simulink model "Tavola3_SIM"  (R2018b)
settings: Solver=VariableStepAuto  StartTime=0.0  StopTime=50  RelTol=1e-3
values from neighbouring files (symbols this model uses):
  cond_iniziali = [0,0,0,10*pi/180,0,5,0]    [tavola3_LAST.m]
  cz = R    (= 0.25)    [tavola3_COORDINATEPENDOLO.m]    (also in tavola3_LAST.m; tavola3_x3x6.m; zero_dyn_x3x6.m)
  K1 = place(A_min,B_min,poles)    [tavola3_COORDINATEPENDOLO.m]    (also in tavola3_LAST.m; tavola3_x3x6.m)
  K2 = place(A_min2,B_min2,poles)    [tavola3_COORDINATEPENDOLO.m]    (also in tavola3_LAST.m; tavola3_x3x6.m)
undefined symbols (not defined in the file or in its folder): sigbuilder_block
libraries: simulink x1
settings Model: Creator=Utente  LastModifiedBy=Utente

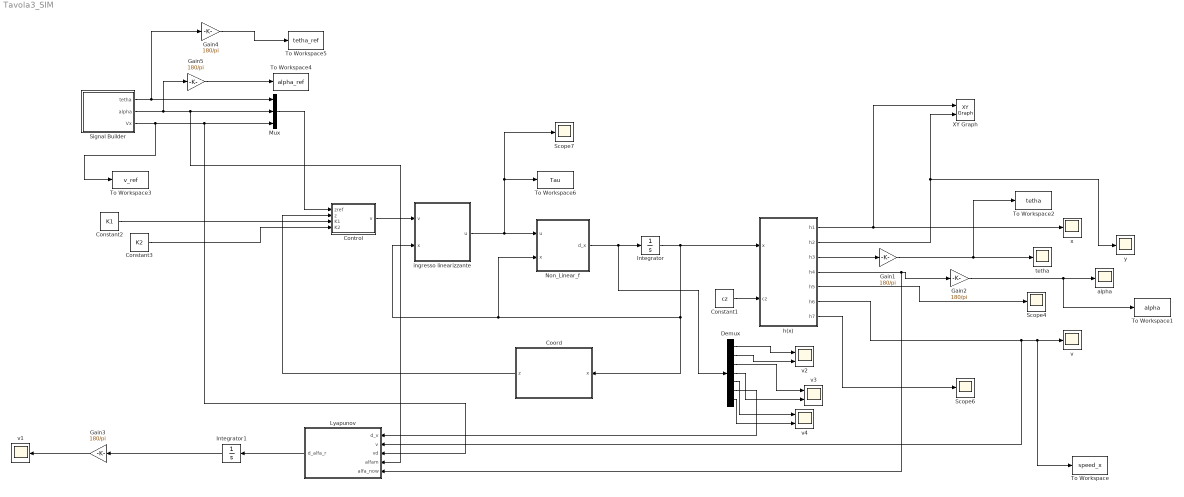
== system Tavola3_SIM ==
  Constant1 : Constant  Value=cz
  Constant2 : Constant  Value=K1
  Constant3 : Constant  Value=K2
  Control : MATLAB Function  TreatAsAtomicUnit=on
  Coord : MATLAB Function  TreatAsAtomicUnit=on
  Demux : Demux  Outputs=7
  Gain{1..5} (5 alike) : Gain  Gain=180/pi
  Integrator : Integrator  InitialCondition=cond_iniziali
  Integrator1 : Integrator
  Lyapunov : MATLAB Function  TreatAsAtomicUnit=on
  Mux : Mux  Inputs=3
  "Non_Linear_f " : MATLAB Function  TreatAsAtomicUnit=on
  Scope4 : Scope
  Scope6 : Scope
  Scope7 : Scope
  Signal Builder : Subsystem  Tag=STV Subsys  LoadFcn=sigbuilder_block('load');  StartFcn=sigbuilder_block('start');  StopFcn=sigbuilder_block('stop');  ClipboardFcn=sigbuilder_block('clipboard');  mask(Sigbuilder block){tuvar=[0:10]}
      mask help: Simulink:masks:SigbuilderBlock_MD
      mask init:
      | if ~strcmp(get_param(bdroot(gcbh),'SimulationStatus'),'stopped') tuvar = sigbuilder_block('maskInit'); end
      settings: CopyFcn=sigbuilder_block('copy');  DeleteFcn=sigbuilder_block('delete');  ModelCloseFcn=sigbuilder_block('modelClose');  PreSaveFcn=sigbuilder_block('preSave');  PauseFcn=sigbuilder_block('pause');  ContinueFcn=sigbuilder_block('continue');  NameChangeFcn=sigbuilder_block('namechange');  OpenFcn=sigbuilder_block('open',[40.5 0 978 477.75 ]);  CloseFcn=sigbuilder_block('close');
      mask Display: plot(0, 0, 100, 100,[2, 2, 32, 32, 2], [68, 8, 8, 68, 68],[32, 2], [38, 38], [32, 19, 2],[53, 60, 44], [32, 17, 17, 2],[16, 16, 31, 31]);txt = getActiveGroup(gcbh);text(2, 100, txt,'verticalAlignment', 'top');
  To Workspace : ToWorkspace  VariableName=speed_x  SaveFormat=Structure With Time  SampleTime=-1
  To Workspace1 : ToWorkspace  VariableName=alpha  SaveFormat=Structure With Time  SampleTime=-1
  To Workspace2 : ToWorkspace  VariableName=tetha  SaveFormat=Structure With Time  SampleTime=-1
  To Workspace3 : ToWorkspace  VariableName=v_ref  SaveFormat=Structure With Time  SampleTime=-1
  To Workspace4 : ToWorkspace  VariableName=alpha_ref  SaveFormat=Structure With Time  SampleTime=-1
  To Workspace5 : ToWorkspace  VariableName=tetha_ref  SaveFormat=Structure With Time  SampleTime=-1
  To Workspace6 : ToWorkspace  VariableName=Tau  SaveFormat=Structure With Time  SampleTime=-1
  XY Graph : simulink/Sinks/XY Graph  xmin=-100  xmax=100  ymin=-100  ymax=100  st=-1
  alpha : Scope
  h(x) : MATLAB Function  TreatAsAtomicUnit=on
  ingresso linearizzante : MATLAB Function  TreatAsAtomicUnit=on
  tetha : Scope
  v : Scope
  v1 : Scope
  v2 : Scope  NumInputPorts=2
  v3 : Scope  NumInputPorts=2
  v4 : Scope  NumInputPorts=2
  x : Scope
  y : Scope
  wires:
  "Non_Linear_f "/1(d_x) -> Demux/1, Integrator/1
  Integrator/1 -> Coord/1(x), ingresso linearizzante/2(x), "Non_Linear_f "/2(x), h(x)/1(x)
  ingresso linearizzante/1(u) -> To Workspace6/1, Scope7/1, "Non_Linear_f "/1(u)
  Control/1(v) -> ingresso linearizzante/1(v)
  h(x)/2(h2) -> XY Graph/2, y/1
  Coord/1(z) -> Control/2(z)
  h(x)/3(h3) -> Gain1/1
  h(x)/5(h5) -> Scope4/1
  Constant1/1 -> h(x)/2(cz)
  Constant2/1 -> Control/3(K1)
  Constant3/1 -> Control/4(K2)
  h(x)/7(h7) -> Scope6/1
  Mux/1 -> Control/1(zref)
  Signal Builder/1(tetha) -> Gain4/1, Mux/1
  h(x)/6(h6) -> Lyapunov/2(v), To Workspace/1, v/1
  h(x)/4(h4) -> Lyapunov/5(alfa_now), Gain2/1
  Gain1/1 -> To Workspace2/1, tetha/1
  h(x)/1(h1) -> x/1, XY Graph/1
  Gain2/1 -> alpha/1, To Workspace1/1
  Lyapunov/1(d_alfa_r) -> Integrator1/1
  Demux/6 -> Lyapunov/1(d_v)
  Signal Builder/2(alpha) -> Gain5/1, Lyapunov/4(alfam), Mux/2
  Integrator1/1 -> Gain3/1
  Gain3/1 -> v1/1
  Signal Builder/3(Vx) -> To Workspace3/1, Lyapunov/3(vd), Mux/3
  Gain4/1 -> To Workspace5/1
  Gain5/1 -> To Workspace4/1
  Demux/1 -> v2/1
  Demux/2 -> v2/2
  Demux/3 -> v3/1
  Demux/4 -> v3/2
  Demux/5 -> v4/1
  Demux/7 -> v4/2

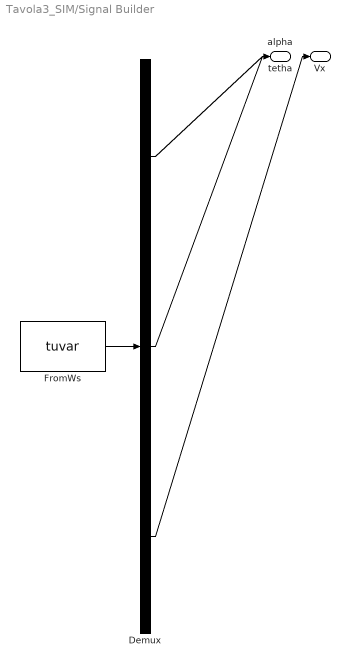
== system Tavola3_SIM/Signal Builder ==
  Demux : Demux  Tag=STV Demux  Outputs=3
  FromWs : FromWorkspace  Tag=STV FromWs  VariableName=tuvar  SampleTime=0
      SigBuilderData=|
      | common.afterFinalStr = 'Extrapolate'
      | common.sampleTime = 0
      | dataSet.timeRange = [0 50]
      | dataSet.name = 'Group 1'
      | sbobj.Groups.Name = 'Group 1'
      | sbobj.Groups.Signals(1).Name = 'tetha'
      | sbobj.Groups.Signals(1).XData = [0 50]
      | sbobj.Groups.Signals(1).YData = [1.57079632679 1.57079632679]
      | sbobj.Groups.Signals(2).Name = 'alpha'
      | sbobj.Groups.Signals(2).XData = [0 5.01 5.01 50]
      | sbobj.Groups.Signals(2).YData = [0.366 0.366 0 0]
      | sbobj.Groups.Signals(3).Name = 'Vx'
      | sbobj.Groups.Signals(3).XData = [0 5.99 20 20 50]
      | sbobj.Groups.Signals(3).YData = [5 4.95 4.9 0 0]
      | sbobj.Groups.TimeRange = [0 50]
  tetha : Outport  Tag=STV Outport
  alpha : Outport  Tag=STV Outport  Port=2
  Vx : Outport  Tag=STV Outport  Port=3
  wires:
  FromWs/1 -> Demux/1
  Demux/1 -> tetha/1
  Demux/2 -> alpha/1
  Demux/3 -> Vx/1

== matlab function Tavola3_SIM/h(x) ==
  data: x input; h1 output; h2 output; h3 output; h4 output; h5 output; h6 output; h7 output; cz input
function [h1,h2,h3,h4,h5,h6,h7] = h(x,cz)

x1 = x(1);
x2 = x(2);
x3 = x(3);
x4 = x(4);
x5 = x(5);
x6 = x(6);
x7 = x(7);

h1 = x1;
h2 = x2;
h3 = x3;
h4 = x4;
h5 = x5;
h6 = x6;
h7 = x7;

== matlab function Tavola3_SIM/Non_Linear_f  ==
  data: u input; d_x output; x input
function d_x = statespacef(u,x)

    x1 = x(1);
    x2 = x(2);
    x3 = x(3);
    x4 = x(4);
    x5 = x(5);
    x6 = x(6);
    x7 = x(7);

    f = [                                                                                                                             x6*cos(x3);                                                                                                                            
                                                                                                                                      x6*sin(x3);
                                                                                                                                              x7;
                                                                                                                                              x5;
     (2.39*sin(2.0*x4)*x5^2)/(4.79*cos(x4)^2 - 12.5) - (267.0*sin(x4))/(4.79*cos(x4)^2 - 12.5) - (3.28*x7^2*sin(2.0*x4))/(4.79*cos(x4)^2 - 12.5);
               (1.99*sin(3.0*x4) - 6.77*sin(x4))*x7^2 + (23.5*sin(2.0*x4))/(4.79*cos(x4)^2 - 12.5) - (2.19*x5^2*sin(x4))/(4.79*cos(x4)^2 - 12.5);
                                           (0.547*x6*x7*sin(x4))/(0.228*cos(x4)^2 - 0.315) + (0.228*x5*x7*sin(2.0*x4))/(0.228*cos(x4)^2 - 0.315)];

    g1_b =   [                                          0;
                                                        0;
                                                        0;
                                                        0;
            (2.19*cos(x4) + 3.11)/(4.79*cos(x4)^2 - 12.5);
     -(1.0*(0.547*cos(x4) + 1.0))/(4.79*cos(x4)^2 - 12.5);
                                                        0];

    g2_b = [                           0;
                                       0;
                                       0;
                                       0;
                                       0;
                                       0;
                 -0.05/(0.228*cos(x4)^2 - 0.315)];

    d_x = f + g1_b*u(1) + g2_b*u(2);
    
end

== matlab function Tavola3_SIM/ingresso linearizzante ==
  data: v input; u output; x input
function u = inputLinearizzante(v,x)

x1 = x(1);
x2 = x(2);
x3 = x(3);
x4 = x(4);
x5 = x(5);
x6 = x(6);
x7 = x(7);

G =  [                                  (0.547*x6*x7*sin(x4))/(0.228*cos(x4)^2 - 0.315) + (0.228*x5*x7*sin(2.0*x4))/(0.228*cos(x4)^2 - 0.315);
 (2.39*sin(2.0*x4)*x5^2)/(4.79*cos(x4)^2 - 12.5) - (267.0*sin(x4))/(4.79*cos(x4)^2 - 12.5) - (3.28*x7^2*sin(2.0*x4))/(4.79*cos(x4)^2 - 12.5)];
 

E = [                                             0, -0.05/(0.228*cos(x4)^2 - 0.315);
     (2.19*cos(x4) + 3.11)/(4.79*cos(x4)^2 - 12.5),                               0];

inv_E = inv(E);

u = -inv_E*G + inv_E*v;

== matlab function Tavola3_SIM/Coord ==
  data: x input; z output
function z = transformCoordinate(x)

    x1 = x(1);
    x2 = x(2);
    x3 = x(3);
    x4 = x(4);
    x5 = x(5);
    x6 = x(6);
    x7 = x(7);

    z = [   x3;
            x7;
            x4;
            x5;
            x1;
            x2;
            x6];
            %-x5*-(1.0*(0.547*cos(x4) + 1.0))/(4.79*cos(x4)^2 - 12.5)+x6*(2.19*cos(x4) + 3.11)/(4.79*cos(x4)^2 - 12.5)];
 %-x5*g1(6) + x6*g1(5)
 

end

== matlab function Tavola3_SIM/Control ==
  data: zref input; z input; v output; K1 input; K2 input
function v = control(zref,z,K1,K2)
    
    v = zeros(2,1);
    
    k = [K1(1),K1(2),0,0,0,0,0;
         0,0,K2(1),K2(2),0,0,0];
         
    v(1) = -(k(1,1)*(z(1)-zref(1)) + k(1,2)*(z(2))) - 5*((z(7)-zref(3)));
    v(2) = -(k(2,3)*(z(3)-zref(2)) + k(2,4)*(z(4))) - 50*((z(7)-zref(3)));
    
end

== matlab function Tavola3_SIM/Lyapunov ==
  data: d_v input; d_alfa_r output; v input; vd input; alfam input; alfa_now input
function d_alfa_r = Lyapunov(d_v,v,vd,alfam,alfa_now)

    
    d_alfa_r = (1/alfa_now*(alfam^2-alfa_now^2)^2)*2*(v-vd);
%     d_alfa_r = -10*(v-vd)*d_v/alfa_now - 20*alfa_now;
    
    
end
